simulink model "env_extQ16"  (R2022b)
settings: Solver=VariableStepAuto  StartTime=0.0  StopTime=30  RelTol=1e-3
values from neighbouring files (symbols this model uses):
  B = 8    [variables.m]    (also in variables16.m)
  cordic_delay = 20    [variables.m]    (also in variables16.m)
  e_val = 1/l2    [variables.m]    (also in variables16.m)
  exp_fract_len_homo = 26    [variables.m]    (also in variables16.m = 10)
  exp_word_len_homo = 32    [variables.m]    (also in variables16.m = 16)
  explarge_delay = 3    [variables.m]    (also in variables16.m)
  fft_len_hilb = 2048    [variables.m]    (also in variables16.m)
  fft_length = 4096    [variables.m]    (also in variables16.m)
  frac_bit_l2 = 30    [variables.m]    (also in variables16.m = 14)
  frac_bit_l3 = 29    [variables.m]    (also in variables16.m = 13)
  frac_bit_l4 = 28    [variables.m]    (also in variables16.m = 12)
  grp_delay_hilb = 11    [variables.m]    (also in variables16.m)
  grp_delay_homo = 13    [variables.m]    (also in variables16.m)
  grp_delay_psd = 19    [variables.m]    (also in variables16.m)
  grp_delay_swt = 12    [variables.m]    (also in variables16.m)
  l2 = log(2)    [variables.m]    (also in variables16.m)
  l2e = 1/log2(exp(1))    [variables.m]    (also in variables16.m)
  log2_table = log2((2^(B-1) : 2^(B)) / 2^(B - 1))    [variables.m]    (also in variables16.m)
  log_fract_len_homo = 31    [variables.m]    (also in variables16.m = 15)
  log_latency = 21    [variables.m]    (also in variables16.m)
  log_word_len = 48    [variables.m]    (also in variables16.m = 24)
  log_word_len_homo = 32    [variables.m]    (also in variables16.m = 16)
  NLZLUT = B-ceil(log2((1:2^B)))    [variables.m]    (also in variables16.m)
  scale = 1.0 / (fs * sum(window_val.*window_val))    [variables.m]    (also in variables16.m)
  win_dim = 64    [variables.m]    (also in variables16.m)
  window_dim = 100    [variables.m]    (also in variables16.m)
undefined symbols (not defined in the file or in its folder): C, c, fl_high_index, fl_low_index, HiD, hilbert_fifo_full, LoD, psd_fifo_full, SFVC784, swt_fifo_full, XCK26, xlfda_numerator
libraries: hdlBasic x626, hdlDSPIP x12, hdlUtilities x2, dspsnks4 x1, dspvision x1, vmcUtilities x1
(part 2 of 7)

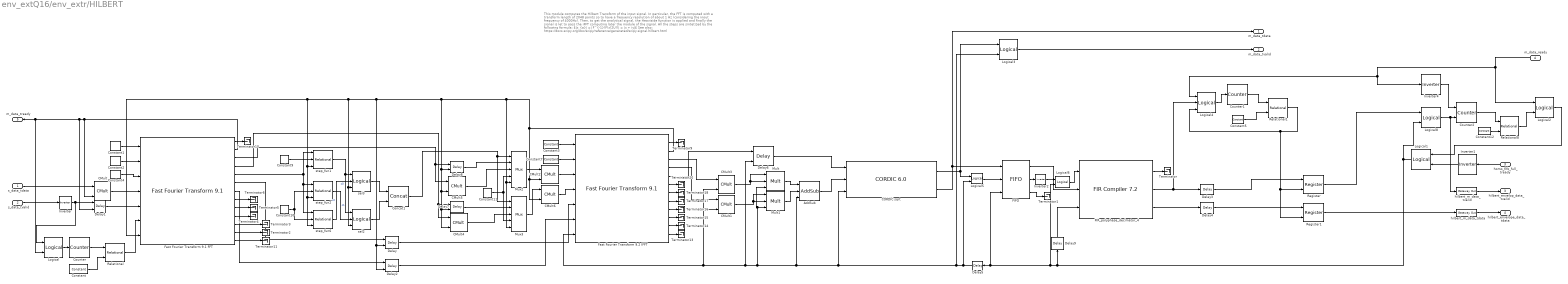
== system env_extQ16/env_extr/HILBERT ==
  note: This module computes the Hilbert Transform of the input signal.
      | In particular, the FFT is computed with a transform length of 2048 points so to have a frequency resolution of about 1 Hz (considering the input frequency of 4000Hz).
      | Then, to get the analytical signal, the Heaviside function is applied and finally the signal is let to pass the iFFT computing later the module of the signal.
      |
      | All the steps are sintetized by the following formula:
      | $|x_{a}| =| F^{-1}(F(x)2U))| = |x + iy|$
      |
      | See also: https://docs.scipy.org/doc/scipy/reference/generated/scipy.signal.hilbert.html
  s_data_tdata : Inport
  s_data_tvalid : Inport  Port=2
  homo_fifo_full_tready : Inport  Port=3
  m_data_ready : Inport  Port=4
  AddSub : hdlBasic/AddSub  mode=Addition  use_carryin=off  use_carryout=off  en=on  latency=1  precision=User Defined  arith_type=Unsigned  n_bits=32  bin_pt=31  quantization="Round  (unbiased: +/- Inf)"  overflow=Wrap  use_behavioral_HDL=off  hw_selection=Fabric  pipelined=off  XmcBlockStatus=1  maskContainerNames=tabcontainer1  block_type=addsub  block_config=sysgen:Addsub_config
  CMult : hdlBasic/CMult  const=1/2  gui_display_data_type=Fixed-point  const_n_bits=32  const_bin_pt=31  float_type=Single  exp_bits=8  fraction_bits=24  en=on  latency=1  precision=User Defined  arith_type="Signed  (2's comp)"  n_bits=34  bin_pt=33  quantization="Round  (unbiased: +/- Inf)"  overflow=Wrap  use_behavioral_HDL=off  mem_type=Distributed RAM  pipeline=off  XmcBlockStatus=1  maskContainerNames=tabcontainer1  block_type=cmult  block_config=sysgen:CMult_config
      settings: infoedit=[]
  CMult1 : hdlBasic/CMult  const=1/fft_len_hilb*128  gui_display_data_type=Fixed-point  const_n_bits=32  const_bin_pt=31  float_type=Single  exp_bits=8  fraction_bits=24  en=on  latency=1  precision=User Defined  arith_type="Signed  (2's comp)"  n_bits=32  bin_pt=30  quantization="Round  (unbiased: +/- Inf)"  overflow=Wrap  use_behavioral_HDL=off  mem_type=Distributed RAM  pipeline=off  XmcBlockStatus=1  maskContainerNames=tabcontainer1  block_type=cmult  block_config=sysgen:CMult_config
      settings: infoedit=[]
  CMult2 : hdlBasic/CMult  const=1/64  gui_display_data_type=Fixed-point  const_n_bits=32  const_bin_pt=31  float_type=Single  exp_bits=8  fraction_bits=24  en=on  latency=1  precision=User Defined  arith_type="Signed  (2's comp)"  n_bits=34  bin_pt=33  quantization="Round  (unbiased: +/- Inf)"  overflow=Wrap  use_behavioral_HDL=off  mem_type=Distributed RAM  pipeline=off  XmcBlockStatus=1  maskContainerNames=tabcontainer1  block_type=cmult  block_config=sysgen:CMult_config
      settings: infoedit=[]
  CMult3 : hdlBasic/CMult  const=1/fft_len_hilb*128  gui_display_data_type=Fixed-point  const_n_bits=32  const_bin_pt=31  float_type=Single  exp_bits=8  fraction_bits=24  en=on  latency=1  precision=User Defined  arith_type="Signed  (2's comp)"  n_bits=32  bin_pt=30  quantization="Round  (unbiased: +/- Inf)"  overflow=Wrap  use_behavioral_HDL=off  mem_type=Distributed RAM  pipeline=off  XmcBlockStatus=1  maskContainerNames=tabcontainer1  block_type=cmult  block_config=sysgen:CMult_config
      settings: infoedit=[]
  CMult4 : hdlBasic/CMult  const=2  gui_display_data_type=Fixed-point  const_n_bits=32  const_bin_pt=30  float_type=Single  exp_bits=8  fraction_bits=24  en=on  latency=2  precision=Full  arith_type="Signed  (2's comp)"  n_bits=16  bin_pt=14  quantization=Truncate  overflow=Wrap  use_behavioral_HDL=off  mem_type=Distributed RAM  pipeline=off  XmcBlockStatus=1  maskContainerNames=tabcontainer1  block_type=cmult  block_config=sysgen:CMult_config
      settings: infoedit=[]
  CMult5 : hdlBasic/CMult  const=2  gui_display_data_type=Fixed-point  const_n_bits=32  const_bin_pt=30  float_type=Single  exp_bits=8  fraction_bits=24  en=on  latency=2  precision=Full  arith_type="Signed  (2's comp)"  n_bits=16  bin_pt=14  quantization=Truncate  overflow=Wrap  use_behavioral_HDL=off  mem_type=Distributed RAM  pipeline=off  XmcBlockStatus=1  maskContainerNames=tabcontainer1  block_type=cmult  block_config=sysgen:CMult_config
      settings: infoedit=[]
  CMult6 : hdlBasic/CMult  const=1/64  gui_display_data_type=Fixed-point  const_n_bits=32  const_bin_pt=31  float_type=Single  exp_bits=8  fraction_bits=24  en=on  latency=1  precision=User Defined  arith_type="Signed  (2's comp)"  n_bits=34  bin_pt=33  quantization="Round  (unbiased: +/- Inf)"  overflow=Wrap  use_behavioral_HDL=off  mem_type=Distributed RAM  pipeline=off  XmcBlockStatus=1  maskContainerNames=tabcontainer1  block_type=cmult  block_config=sysgen:CMult_config
      settings: infoedit=[]
  CORDIC sqrt : hdlDSPIP/CORDIC 6.0   functional_selection=Square_Root  architectural_configuration=Parallel  pipelining_mode=Maximum  data_format=UnsignedFraction  phase_format=Radians  input_width=32  output_width=32  round_mode=Nearest_Even  iterations=0  precision=0  compensation_scaling=No_Scale_Compensation  coarse_rotation=off  aclken=on  aresetn=off  out_tready=off  cartesian_has_tuser=off  cartesian_has_tlast=off  cartesian_tuser_width=1  phase_has_tuser=off  phase_has_tlast=off  phase_tuser_width=1  out_tlast_behv=Null  flow_control=NonBlocking  optimize_goal=Resources  trim_axipin_name=off  simulation_type=hybrid_sim  simulation_model=sysgen:cordic_v6_0  data_path_portlist={'s_axis_cartesian_tdata_imag', 's_axis_cartesian_tdata_real', 's_axis_phase_tdata_phase', 'm_axis_dout_tdata_imag', 'm_axis_dout_tdata_real', 'm_axis_dout_tdata_phase','m_axis_dout_tdata'}  ip_name=CORDIC  ip_version=6.0  dsptool_ready=true  ipcore_usecache=true  ipcore_useipmodelcache=true  wrapper_available=true  port_translation_map={ 'aclken' => 'en', 'aresetn' => 'rst' }  XmcBlockStatus=1  maskContainerNames=group15  block_type=cordic_v6_0  block_config=sysgen:rodinimport_config  block_width=800
  Concat1 : hdlBasic/Concat  num_inputs=2  XmcBlockStatus=1  maskContainerNames=group1  block_type=concat  block_config=sysgen:Concat_config
  Constant : hdlBasic/Constant  const=fft_len_hilb-1  gui_display_data_type=Fixed-point  arith_type=Signed (2's comp)  n_bits=log2(fft_len_hilb)+1  bin_pt=0  preci_type=Single  exp_width=8  frac_width=24  explicit_period=off  period=1  XmcBlockStatus=1  maskContainerNames=tabcontainer1  block_type=constant  block_config=sysgen:Constant_config
  Constant1 : hdlBasic/Constant  const=1.0  gui_display_data_type=Fixed-point  arith_type=Unsigned  n_bits=1  bin_pt=0  preci_type=Single  exp_width=8  frac_width=24  explicit_period=off  period=1  XmcBlockStatus=1  maskContainerNames=tabcontainer1  block_type=constant  block_config=sysgen:Constant_config
  Constant10 : hdlBasic/Constant  const=fft_len_hilb/2  gui_display_data_type=Fixed-point  arith_type=Unsigned  n_bits=ceil(log2(fft_len_hilb/2+1))  bin_pt=0  preci_type=Single  exp_width=8  frac_width=24  explicit_period=on  period=sample_period_hilbert  XmcBlockStatus=1  maskContainerNames=tabcontainer1  block_type=constant  block_config=sysgen:Constant_config
  Constant11 : hdlBasic/Constant  const=0  gui_display_data_type=Fixed-point  arith_type=Signed (2's comp)  n_bits=16  bin_pt=14  preci_type=Single  exp_width=8  frac_width=24  explicit_period=off  period=1  XmcBlockStatus=1  maskContainerNames=tabcontainer1  block_type=constant  block_config=sysgen:Constant_config
  Constant12 : hdlBasic/Constant  const=win_dim  gui_display_data_type=Fixed-point  arith_type=Unsigned  n_bits=win_bit  bin_pt=0  preci_type=Single  exp_width=8  frac_width=24  explicit_period=off  period=1  XmcBlockStatus=1  maskContainerNames=tabcontainer1  block_type=constant  block_config=sysgen:Constant_config
  Constant2 : hdlBasic/Constant  const=1.0  gui_display_data_type=Boolean  arith_type=Boolean  n_bits=1  bin_pt=0  preci_type=Single  exp_width=8  frac_width=24  explicit_period=off  period=1  XmcBlockStatus=1  maskContainerNames=tabcontainer1  block_type=constant  block_config=sysgen:Constant_config
  Constant3 : hdlBasic/Constant  const=0  gui_display_data_type=Fixed-point  arith_type=Unsigned  n_bits=1  bin_pt=0  preci_type=Single  exp_width=8  frac_width=24  explicit_period=off  period=1  XmcBlockStatus=1  maskContainerNames=tabcontainer1  block_type=constant  block_config=sysgen:Constant_config
  Constant4 : hdlBasic/Constant  const=0  gui_display_data_type=Fixed-point  arith_type=Signed (2's comp)  n_bits=34  bin_pt=33  preci_type=Single  exp_width=8  frac_width=24  explicit_period=on  period=sample_period_hilbert  XmcBlockStatus=1  maskContainerNames=tabcontainer1  block_type=constant  block_config=sysgen:Constant_config
  Constant5 : hdlBasic/Constant  const=grp_delay_hilb  gui_display_data_type=Fixed-point  arith_type=Unsigned  n_bits=ceil(log2(grp_delay_hilb))  bin_pt=0  preci_type=Single  exp_width=8  frac_width=24  explicit_period=off  period=1  XmcBlockStatus=1  maskContainerNames=tabcontainer1  block_type=constant  block_config=sysgen:Constant_config
  Constant7 : hdlBasic/Constant  const=1.0  gui_display_data_type=Boolean  arith_type=Boolean  n_bits=1  bin_pt=0  preci_type=Single  exp_width=8  frac_width=24  explicit_period=off  period=1  XmcBlockStatus=1  maskContainerNames=tabcontainer1  block_type=constant  block_config=sysgen:Constant_config
  Constant9 : hdlBasic/Constant  const=0  gui_display_data_type=Fixed-point  arith_type=Unsigned  n_bits=1  bin_pt=0  preci_type=Single  exp_width=8  frac_width=24  explicit_period=on  period=sample_period_hilbert  XmcBlockStatus=1  maskContainerNames=tabcontainer1  block_type=constant  block_config=sysgen:Constant_config
  Counter : hdlBasic/Counter  cnt_type=Free running  cnt_to=Inf  operation=Up  start_count=0  cnt_by_val=1  arith_type=Unsigned  n_bits=11  bin_pt=0  load_pin=off  rst=off  en=on  explicit_period=Explicit  period=sample_period_hilbert  use_behavioral_HDL=off  implementation=Fabric  XmcBlockStatus=1  maskContainerNames=group1  block_type=counter  block_config=sysgen:Counter_config  block_width=531  block_height=1023
  Counter1 : hdlBasic/Counter  cnt_type=Free running  cnt_to=Inf  operation=Up  start_count=0  cnt_by_val=1  arith_type=Unsigned  n_bits=ceil(log2(grp_delay_hilb))  bin_pt=0  load_pin=off  rst=off  en=on  explicit_period=Explicit  period=sample_period_hilbert  use_behavioral_HDL=off  implementation=Fabric  XmcBlockStatus=1  maskContainerNames=group1  block_type=counter  block_config=sysgen:Counter_config  block_width=531  block_height=1023
  Counter2 : hdlBasic/Counter  cnt_type=Free running  cnt_to=Inf  operation=Up  start_count=0  cnt_by_val=1  arith_type=Unsigned  n_bits=win_bit  bin_pt=0  load_pin=off  rst=on  en=on  explicit_period=Explicit  period=sample_period_psd  use_behavioral_HDL=off  implementation=Fabric  XmcBlockStatus=1  maskContainerNames=group1  block_type=counter  block_config=sysgen:Counter_config  block_width=531  block_height=1023
  Delay : hdlBasic/Delay  rst=off  en=on  latency=4  reg_retiming=off  XmcBlockStatus=1  maskContainerNames=group1  block_type=delay  block_config=sysgen:Delay_config
  Delay1 : hdlBasic/Delay  rst=off  en=on  latency=1  reg_retiming=off  XmcBlockStatus=1  maskContainerNames=group1  block_type=delay  block_config=sysgen:Delay_config
  Delay2 : hdlBasic/Delay  rst=off  en=on  latency=4  reg_retiming=off  XmcBlockStatus=1  maskContainerNames=group1  block_type=delay  block_config=sysgen:Delay_config
  Delay3 : hdlBasic/Delay  rst=off  en=off  latency=1  reg_retiming=off  XmcBlockStatus=1  maskContainerNames=group1  block_type=delay  block_config=sysgen:Delay_config
  Delay4 : hdlBasic/Delay  rst=off  en=off  latency=1  reg_retiming=off  XmcBlockStatus=1  maskContainerNames=group1  block_type=delay  block_config=sysgen:Delay_config
  Delay5 : hdlBasic/Delay  rst=off  en=off  latency=64*(grp_delay_homo-grp_delay_hilb)  reg_retiming=off  XmcBlockStatus=1  maskContainerNames=group1  block_type=delay  block_config=sysgen:Delay_config
  Delay6 : hdlBasic/Delay  rst=off  en=on  latency=5  reg_retiming=off  XmcBlockStatus=1  maskContainerNames=group1  block_type=delay  block_config=sysgen:Delay_config
  Delay7 : hdlBasic/Delay  rst=off  en=on  latency=2  reg_retiming=off  XmcBlockStatus=1  maskContainerNames=group1  block_type=delay  block_config=sysgen:Delay_config
  Delay8 : hdlBasic/Delay  rst=off  en=on  latency=2  reg_retiming=off  XmcBlockStatus=1  maskContainerNames=group1  block_type=delay  block_config=sysgen:Delay_config
  Delay9 : hdlBasic/Delay  rst=off  en=off  latency=1  reg_retiming=off  XmcBlockStatus=1  maskContainerNames=group1  block_type=delay  block_config=sysgen:Delay_config
  FIFO : hdlBasic/FIFO  mem_type=Block RAM  performance_options=Standard_FIFO  embedded_registers=off  depth=256  use_asym_data_widths=off  asym_read_width=32  percent_nbits=1  rst=off  rst_latency=2  en=off  use_dcount=off  use_percent_full_port=off  use_almost_empty=off  almost_empty_thresh=2  use_almost_full=off  use_rd_rst_busy=off  use_wr_rst_busy=off  almost_full_thresh=14  almost_empty_offset=[]  almost_full_offset=[]  explicit_period=off  period=[]  store_only_valid=[]  init_zero=[]  simulation_type=fast_sim  XmcBlockStatus=1  maskContainerNames=tabcontainer1  block_type=fifo  block_config=sysgen:FIFO_config  block_width=538  block_height=997
      settings: infoedit=[]
  FIR_polyphase_decimator_4 : hdlDSPIP/FIR Compiler 7.2   coefficientvector=firdecim.Numerator  coefficient_sets=1  coefficient_reload=off  filter_type=Decimation  rate_change_type=Integer  interpolation_rate=1  decimation_rate=80  zero_pack_factor=1  channel_sequence=Basic  number_channels=1  pattern_list='P4-0,P4-1,P4-2,P4-3,P4-4'  number_paths=1  ratespecification=Input_Sample_Period  sampleperiod=1.00000000  hardwareoversamplingrate=1  coefficient_sign=Signed  quantization=Quantize_Only  coefficient_width=coeff_width  bestprecision=on  coefficient_fractional_bits=37  coefficient_structure=Non_Symmetric  output_rounding_mode=Convergent_Rounding_to_Even  output_width=32  filter_architecture=Systolic_Multiply_Accumulate  optimization_goal=Area  optimization_list='None'  data_buffer_type=Automatic  coefficient_buffer_type=Automatic  input_buffer_type=Automatic  output_buffer_type=Automatic  preference_for_other_storage=Automatic  multi_column_support=Automatic  columnconfig='24'  inter_column_pipe_length=4  data_has_tlast=Not_Required  m_data_has_tready=off  s_data_has_fifo=off  s_data_has_tuser=Not_Required  m_data_has_tuser=Not_Required  s_config_sync_mode=On_Vector  s_config_method=Single  num_reload_slots=1  has_aclken=on  has_aresetn=off  reset_data_vector=on  trim_axipin_name=off  simulation_type=hybrid_sim  simulation_model=sysgen:xfirv7_2_cmodel  data_path_portlist={ 's_axis_data_tdata', 'm_axis_data_tdata' }  passband_min=0.0  passband_max=0.5  stopband_min=0.5  stopband_max=1.0  filter_selection=1  gui_behaviour='Sysgen_GUI'  data_sign=Signed  data_width=16  data_fractional_bits=0  data_tuser_width=1  wrapper_available=true  ip_wrap_arbitrary_binary_point=true  ip_name=FIR Compiler  ip_version=7.2  dsptool_ready=true  ipcore_usecache=true  ipcore_useipmodelcache=true  port_translation_map={ 'aclken' => 'en', 'aresetn' => 'rst' }  run_core_at_system_period=true  ipcore_xco_need_fpga_part=true  ipcore_fpga_part=[]  XmcBlockStatus=1  maskContainerNames=tabcontainer1  block_type=fir_compiler_v7_2  block_config=sysgen:rodinimport_config  block_width=820  block_height=600
  Fast Fourier Transform 9.1 FFT : hdlDSPIP/Fast Fourier Transform 9.1   transform_length=2048  target_clock_frequency=fft_freq  target_data_throughput=50  implementation_options=radix_2_burst_io  run_time_configurable_transform_length=off  phase_factor_width=33  scaling_options=unscaled  rounding_modes=convergent_rounding  aclken=off  aresetn=off  output_ordering=natural_order  cyclic_prefix_insertion=off  throttle_scheme=nonrealtime  xk_index=on  ovflo=off  trim_axipin_name=off  memory_options_data=block_ram  memory_options_phase_factors=block_ram  number_of_stages_using_block_ram_for_data_and_phase_factors=6  memory_options_reorder=block_ram  memory_options_hybrid=off  complex_mult_type=use_mults_resources  butterfly_type=use_luts  simulation_type=hybrid_sim  simulation_model=sysgen:xfftv9_cmodel  data_path_portlist={ 's_axis_data_tdata', 'm_axis_data_tdata', 'm_axis_status_tdata', 'event_fft_overflow' }  channels=1  input_ordering=natural_order  input_width=16  ip_name=Fast Fourier Transform  ip_version=9.1  dsptool_ready=true  ipcore_usecache=true  ipcore_useipmodelcache=true  wrapper_available=true  port_translation_map={ 'aclken' => 'en', 'aresetn' => 'rst'}  data_format=fixed_point  XmcBlockStatus=1  maskContainerNames=tabcontainer1  block_type=xfft_v9_1  block_config=sysgen:rodinimport_config
  Fast Fourier Transform 9.2 IFFT : hdlDSPIP/Fast Fourier Transform 9.1   transform_length=2048  target_clock_frequency=fft_freq  target_data_throughput=50  implementation_options=radix_2_burst_io  run_time_configurable_transform_length=off  phase_factor_width=33  scaling_options=unscaled  rounding_modes=convergent_rounding  aclken=off  aresetn=off  output_ordering=natural_order  cyclic_prefix_insertion=off  throttle_scheme=nonrealtime  xk_index=off  ovflo=off  trim_axipin_name=off  memory_options_data=block_ram  memory_options_phase_factors=block_ram  number_of_stages_using_block_ram_for_data_and_phase_factors=6  memory_options_reorder=block_ram  memory_options_hybrid=off  complex_mult_type=use_mults_resources  butterfly_type=use_luts  simulation_type=hybrid_sim  simulation_model=sysgen:xfftv9_cmodel  data_path_portlist={ 's_axis_data_tdata', 'm_axis_data_tdata', 'm_axis_status_tdata', 'event_fft_overflow' }  channels=1  input_ordering=natural_order  input_width=16  ip_name=Fast Fourier Transform  ip_version=9.1  dsptool_ready=true  ipcore_usecache=true  ipcore_useipmodelcache=true  wrapper_available=true  port_translation_map={ 'aclken' => 'en', 'aresetn' => 'rst'}  data_format=fixed_point  XmcBlockStatus=1  maskContainerNames=tabcontainer1  block_type=xfft_v9_1  block_config=sysgen:rodinimport_config
  Inverter{,1..2,4} (4 alike) : hdlBasic/Inverter  en=off  latency=0  XmcBlockStatus=1  maskContainerNames=group2  block_type=inv  block_config=sysgen:Inverter_config
  Logical{,1..3,5..6,8} (7 alike) : hdlBasic/Logical  logical_function=AND  inputs=2  en=off  latency=0  precision=Full  arith_type=Unsigned  n_bits=16  bin_pt=0  align_bp=on  overflow=[]  quantization=[]  XmcBlockStatus=1  maskContainerNames=tabcontainer1  block_type=logical  block_config=sysgen:Logical_config
  Logical4 : hdlBasic/Logical  logical_function=AND  inputs=3  en=off  latency=0  precision=Full  arith_type=Unsigned  n_bits=16  bin_pt=0  align_bp=on  overflow=[]  quantization=[]  XmcBlockStatus=1  maskContainerNames=tabcontainer1  block_type=logical  block_config=sysgen:Logical_config
  Mult : hdlBasic/Mult  precision=User Defined  arith_type="Signed  (2's comp)"  n_bits=32  bin_pt=31  quantization="Round  (unbiased: +/- Inf)"  overflow=Wrap  en=on  latency=3  use_behavioral_HDL=off  opt=Speed  use_embedded=on  optimum_pipeline=off  pipeline=on  use_rpm=on  placement_style=Triangular  XmcBlockStatus=1  maskContainerNames=group1  block_type=mult  block_config=sysgen:Mult_config  block_width=598  block_height=876
  Mult1 : hdlBasic/Mult  precision=User Defined  arith_type="Signed  (2's comp)"  n_bits=32  bin_pt=31  quantization="Round  (unbiased: +/- Inf)"  overflow=Wrap  en=on  latency=3  use_behavioral_HDL=off  opt=Speed  use_embedded=on  optimum_pipeline=off  pipeline=on  use_rpm=on  placement_style=Triangular  XmcBlockStatus=1  maskContainerNames=group1  block_type=mult  block_config=sysgen:Mult_config  block_width=598  block_height=876
  Mux2 : hdlBasic/Mux  inputs=3  en=on  latency=1  precision=Full  arith_type="Signed  (2's comp)"  n_bits=34  bin_pt=26  quantization="Round  (unbiased: +/- Inf)"  overflow=Wrap  XmcBlockStatus=1  maskContainerNames=tabcontainer1  block_type=mux  block_config=sysgen:Mux_config
  Mux3 : hdlBasic/Mux  inputs=3  en=on  latency=1  precision=Full  arith_type="Signed  (2's comp)"  n_bits=34  bin_pt=26  quantization="Round  (unbiased: +/- Inf)"  overflow=Wrap  XmcBlockStatus=1  maskContainerNames=tabcontainer1  block_type=mux  block_config=sysgen:Mux_config
  Register : hdlBasic/Register  init=0  rst=on  en=off  XmcBlockStatus=1  maskContainerNames=tabcontainer1  block_type=register  block_config=sysgen:Register_config
  Register1 : hdlBasic/Register  init=0  rst=on  en=off  XmcBlockStatus=1  maskContainerNames=tabcontainer1  block_type=register  block_config=sysgen:Register_config
  Relational : hdlBasic/Relational  mode=a=b  op_type=Bool  en=off  latency=1  XmcBlockStatus=1  maskContainerNames=tabcontainer1  block_type=relational  block_config=sysgen:Relational_config
  Relational1 : hdlBasic/Relational  mode=a<b  op_type=Bool  en=off  latency=0  XmcBlockStatus=1  maskContainerNames=tabcontainer1  block_type=relational  block_config=sysgen:Relational_config
  Relational8 : hdlBasic/Relational  mode=a<b  op_type=Bool  en=off  latency=0  XmcBlockStatus=1  maskContainerNames=tabcontainer1  block_type=relational  block_config=sysgen:Relational_config
  Terminator{,1..6,9..11,13..18,20} (17 alike) : Terminator
  hilbert_m_data_tdata : hdlBasic/Gateway Out  inherit_from_input=off  hdl_port=on  rows=1  columns=1  UseAsDAC=off  DACChannel='1'  interface=None  automatic_assignment=on  address_offset=hex2dec('00')  intf_name=''  intf_description=''  timing_constraint=None  locs_specified=off  LOCs={}  io_standard={}  XmcBlockStatus=1  maskContainerNames=group4  block_type=gatewayout  block_config=sysgen:gateway_out_config  block_width_w=590  block_height_w=620  block_width=620  block_height=750
  hilbert_m_data_tvalid : hdlBasic/Gateway Out  inherit_from_input=off  hdl_port=on  rows=1  columns=1  UseAsDAC=off  DACChannel='1'  interface=None  automatic_assignment=on  address_offset=hex2dec('00')  intf_name=''  intf_description=''  timing_constraint=None  locs_specified=off  LOCs={}  io_standard={}  XmcBlockStatus=1  maskContainerNames=group4  block_type=gatewayout  block_config=sysgen:gateway_out_config  block_width_w=590  block_height_w=620  block_width=620  block_height=750
  sel2 : hdlBasic/Logical  logical_function=AND  inputs=2  en=on  latency=1  precision=Full  arith_type=Unsigned  n_bits=16  bin_pt=0  align_bp=on  overflow=[]  quantization=[]  XmcBlockStatus=1  maskContainerNames=tabcontainer1  block_type=logical  block_config=sysgen:Logical_config
  sel3 : hdlBasic/Logical  logical_function=AND  inputs=2  en=on  latency=1  precision=Full  arith_type=Unsigned  n_bits=16  bin_pt=0  align_bp=on  overflow=[]  quantization=[]  XmcBlockStatus=1  maskContainerNames=tabcontainer1  block_type=logical  block_config=sysgen:Logical_config
  step_fun1 : hdlBasic/Relational  mode=a!=b  op_type=Bool  en=on  latency=1  XmcBlockStatus=1  maskContainerNames=tabcontainer1  block_type=relational  block_config=sysgen:Relational_config
  step_fun2 : hdlBasic/Relational  mode=a<b  op_type=Bool  en=on  latency=1  XmcBlockStatus=1  maskContainerNames=tabcontainer1  block_type=relational  block_config=sysgen:Relational_config
  step_fun6 : hdlBasic/Relational  mode=a>b  op_type=Bool  en=on  latency=1  XmcBlockStatus=1  maskContainerNames=tabcontainer1  block_type=relational  block_config=sysgen:Relational_config
  m_data_tdata : Outport
  m_data_tvalid : Outport  Port=2
  hilbert_envelop_data_tvalid : Outport  Port=3
  hilbert_envelope_data_tdata : Outport  Port=4
  m_data_tready : Outport  Port=5
  wires:
  Constant4/1 -> Fast Fourier Transform 9.1 FFT/3
  Constant1/1 -> Fast Fourier Transform 9.1 FFT/1
  Fast Fourier Transform 9.1 FFT/9 -> Terminator5/1
  Fast Fourier Transform 9.1 FFT/8 -> Terminator6/1
  Fast Fourier Transform 9.1 FFT/10 -> Terminator4/1
  Fast Fourier Transform 9.1 FFT/12 -> Terminator2/1
  Fast Fourier Transform 9.1 FFT/1 -> Terminator10/1
  Fast Fourier Transform 9.1 FFT/13 -> Terminator11/1
  Relational/1 -> Fast Fourier Transform 9.1 FFT/6
  Fast Fourier Transform 9.2 IFFT/10 -> Terminator15/1
  Fast Fourier Transform 9.2 IFFT/11 -> Terminator14/1
  Fast Fourier Transform 9.2 IFFT/12 -> Terminator13/1
  Constant7/1 -> Fast Fourier Transform 9.2 IFFT/2
  Fast Fourier Transform 9.2 IFFT/1 -> Terminator9/1
  Fast Fourier Transform 9.2 IFFT/7 -> Terminator18/1
  Delay/1 -> Fast Fourier Transform 9.2 IFFT/5
  Fast Fourier Transform 9.2 IFFT/5 -> Delay6/1
  Fast Fourier Transform 9.2 IFFT/6 -> Terminator20/1
  Fast Fourier Transform 9.2 IFFT/4 -> CMult1/1
  CMult3/1 -> Mult/2, Mult/1
  Fast Fourier Transform 9.2 IFFT/3 -> CMult3/1
  Constant11/1 -> Mux2/4, Mux3/4
  Delay7/1 -> Mux3/2
  CMult5/1 -> Mux2/3
  Delay8/1 -> Mux2/2
  CMult4/1 -> Mux3/3
  Mux3/1 -> CMult6/1
  Mux2/1 -> CMult2/1
  sel2/1 -> Concat1/2
  step_fun1/1 -> sel2/1, sel3/1  "c0"
  Constant10/1 -> step_fun2/2, step_fun6/2
  step_fun6/1 -> sel3/2  "c2"
  sel3/1 -> Concat1/1
  Constant9/1 -> step_fun1/2
  Fast Fourier Transform 9.1 FFT/5 -> step_fun6/1, step_fun2/1, step_fun1/1
  step_fun2/1 -> sel2/2  "c1"
  Concat1/1 -> Mux2/1, Mux3/1
  hilbert_m_data_tdata/1 -> hilbert_envelope_data_tdata/1
  Constant2/1 -> Fast Fourier Transform 9.1 FFT/2
  s_data_tdata/1 -> CMult/1
  Constant3/1 -> Fast Fourier Transform 9.2 IFFT/1
  s_data_tvalid/1 -> Inverter/1
  CMult6/1 -> Fast Fourier Transform 9.2 IFFT/4
  CMult2/1 -> Fast Fourier Transform 9.2 IFFT/3
  FIR_polyphase_decimator_4/2 -> Logical4/2, Delay3/1
  FIR_polyphase_decimator_4/3 -> Delay4/1
  Delay2/1 -> Fast Fourier Transform 9.2 IFFT/6
  Fast Fourier Transform 9.1 FFT/7 -> Delay2/1
  Counter/1 -> Relational/1
  Constant/1 -> Relational/2
  Logical/1 -> Counter/1
  Fast Fourier Transform 9.2 IFFT/8 -> Terminator17/1
  Fast Fourier Transform 9.2 IFFT/9 -> Terminator16/1
  CMult1/1 -> Mult1/1, Mult1/2
  Mult/1 -> AddSub/1
  Mult1/1 -> AddSub/2
  homo_fifo_full_tready/1 -> Inverter1/1
  AddSub/1 -> CORDIC sqrt/2
  Delay6/1 -> CORDIC sqrt/1
  CMult/1 -> Fast Fourier Transform 9.1 FFT/4
  Delay1/1 -> Fast Fourier Transform 9.1 FFT/5
  Inverter/1 -> Logical/1, Delay1/1
  Counter2/1 -> Relational8/1
  Inverter4/1 -> Counter2/1
  Constant12/1 -> Relational8/2
  hilbert_m_data_tvalid/1 -> hilbert_envelop_data_tvalid/1
  Logical8/1 -> hilbert_m_data_tvalid/1, Counter2/2
  CORDIC sqrt/1 -> Logical3/1, Logical5/1
  m_data_ready/1 -> Logical4/1, Inverter4/1, Logical2/1
  Fast Fourier Transform 9.2 IFFT/2 -> CMult6/2, CMult2/2, Mux3/5, Mux2/5, CMult4/2, Delay7/2, CMult5/2, Delay8/2, Delay2/2, Delay/2, sel2/3, sel3/3, step_fun2/3, step_fun6/3, step_fun1/3, Fast Fourier Transform 9.1 FFT/7
  Logical1/1 -> Logical8/2, Delay5/1, FIFO/3, Logical6/2, Delay9/1
  Fast Fourier Transform 9.1 FFT/2 -> m_data_tready/1, Logical/2, Delay1/2, CMult/2
  Fast Fourier Transform 9.1 FFT/6 -> Delay/1
  Fast Fourier Transform 9.1 FFT/4 -> CMult4/1, Delay7/1
  Fast Fourier Transform 9.1 FFT/3 -> CMult5/1, Delay8/1
  Fast Fourier Transform 9.1 FFT/11 -> Terminator3/1
  Inverter1/1 -> Logical1/2
  Logical3/1 -> m_data_tvalid/1
  CORDIC sqrt/2 -> m_data_tdata/1, FIFO/1
  Relational8/1 -> Logical2/2
  Logical2/1 -> Logical1/1
  FIR_polyphase_decimator_4/1 -> Terminator/1
  Counter1/1 -> Relational1/1
  Logical4/1 -> Counter1/1
  Relational1/1 -> Register/2, Register1/2, Logical4/3
  Constant5/1 -> Relational1/2
  Delay3/1 -> Register/1
  Delay4/1 -> Register1/1
  Register/1 -> Logical8/1
  Register1/1 -> hilbert_m_data_tdata/1
  FIFO/2 -> Inverter2/1
  FIFO/3 -> Terminator1/1
  Delay5/1 -> Logical5/2, Logical3/2, CORDIC sqrt/3, AddSub/3, Mult/3, Mult1/3, Delay6/2, Fast Fourier Transform 9.2 IFFT/7, CMult1/2, CMult3/2
  Delay9/1 -> FIR_polyphase_decimator_4/3
  Logical5/1 -> FIFO/2
  FIFO/1 -> FIR_polyphase_decimator_4/2
  Inverter2/1 -> Logical6/1
  Logical6/1 -> FIR_polyphase_decimator_4/1

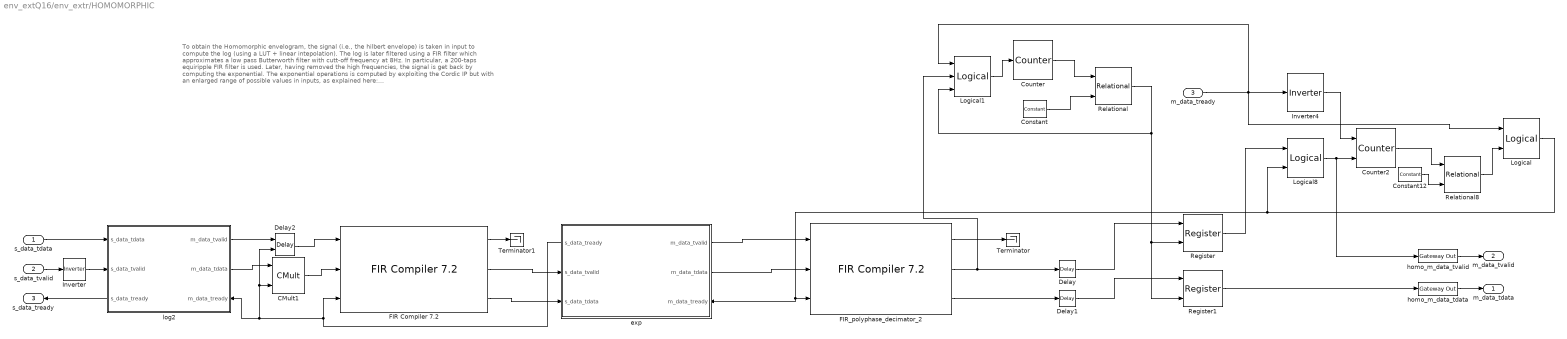
== system env_extQ16/env_extr/HOMOMORPHIC ==
  note: To obtain the Homomorphic envelogram, the signal (i.e., the hilbert envelope) is taken in input to compute the log (using a LUT + linear intepolation).
      |
      | The log is later filtered using a FIR filter which approximates a low pass Butterworth filter with cutt-off frequency at 8Hz. In particular, a 200-taps equiripple FIR filter is used.
      |
      | Later, having removed the high frequencies, the signal is get back by computing the exponential. The exponential operations is computed by exploiting the Cordic IP but with an enlarged range of possible values in inputs, as explained here: https://ieeexplore.ieee.org/document/9012611 .
  s_data_tdata : Inport
  s_data_tvalid : Inport  Port=2
  m_data_tready : Inport  Port=3
  CMult1 : hdlBasic/CMult  const=l2e  gui_display_data_type=Fixed-point  const_n_bits=32  const_bin_pt=31  float_type=Single  exp_bits=8  fraction_bits=24  en=on  latency=1  precision=User Defined  arith_type="Signed  (2's comp)"  n_bits=32  bin_pt=26  quantization="Round  (unbiased: +/- Inf)"  overflow=Saturate  use_behavioral_HDL=off  mem_type=Distributed RAM  pipeline=off  XmcBlockStatus=1  maskContainerNames=tabcontainer1  block_type=cmult  block_config=sysgen:CMult_config
      settings: infoedit=[]
  Constant : hdlBasic/Constant  const=grp_delay_homo  gui_display_data_type=Fixed-point  arith_type=Unsigned  n_bits=ceil(log2(grp_delay_homo))  bin_pt=0  preci_type=Single  exp_width=8  frac_width=24  explicit_period=off  period=1  XmcBlockStatus=1  maskContainerNames=tabcontainer1  block_type=constant  block_config=sysgen:Constant_config
  Constant12 : hdlBasic/Constant  const=win_dim  gui_display_data_type=Fixed-point  arith_type=Unsigned  n_bits=win_bit  bin_pt=0  preci_type=Single  exp_width=8  frac_width=24  explicit_period=off  period=1  XmcBlockStatus=1  maskContainerNames=tabcontainer1  block_type=constant  block_config=sysgen:Constant_config
  Counter : hdlBasic/Counter  cnt_type=Free running  cnt_to=Inf  operation=Up  start_count=0  cnt_by_val=1  arith_type=Unsigned  n_bits=ceil(log2(grp_delay_homo))  bin_pt=0  load_pin=off  rst=off  en=on  explicit_period=Explicit  period=sample_period_homo  use_behavioral_HDL=off  implementation=Fabric  XmcBlockStatus=1  maskContainerNames=group1  block_type=counter  block_config=sysgen:Counter_config  block_width=531  block_height=1023
  Counter2 : hdlBasic/Counter  cnt_type=Free running  cnt_to=Inf  operation=Up  start_count=0  cnt_by_val=1  arith_type=Unsigned  n_bits=win_bit  bin_pt=0  load_pin=off  rst=on  en=on  explicit_period=Explicit  period=sample_period_psd  use_behavioral_HDL=off  implementation=Fabric  XmcBlockStatus=1  maskContainerNames=group1  block_type=counter  block_config=sysgen:Counter_config  block_width=531  block_height=1023
  Delay : hdlBasic/Delay  rst=off  en=off  latency=1  reg_retiming=off  XmcBlockStatus=1  maskContainerNames=group1  block_type=delay  block_config=sysgen:Delay_config
  Delay1 : hdlBasic/Delay  rst=off  en=off  latency=1  reg_retiming=off  XmcBlockStatus=1  maskContainerNames=group1  block_type=delay  block_config=sysgen:Delay_config
  Delay2 : hdlBasic/Delay  rst=off  en=on  latency=1  reg_retiming=off  XmcBlockStatus=1  maskContainerNames=group1  block_type=delay  block_config=sysgen:Delay_config
  FIR Compiler 7.2 : hdlDSPIP/FIR Compiler 7.2   coefficientvector=NUM  coefficient_sets=1  coefficient_reload=off  filter_type=Single_Rate  rate_change_type=Integer  interpolation_rate=1  decimation_rate=1  zero_pack_factor=1  channel_sequence=Basic  number_channels=1  pattern_list='P4-0,P4-1,P4-2,P4-3,P4-4'  number_paths=1  ratespecification=Input_Sample_Period  sampleperiod=1  hardwareoversamplingrate=1  coefficient_sign=Signed  quantization=Quantize_Only  coefficient_width=coeff_width  bestprecision=on  coefficient_fractional_bits=36  coefficient_structure=Symmetric  output_rounding_mode=Convergent_Rounding_to_Even  output_width=output_width  filter_architecture=Systolic_Multiply_Accumulate  optimization_goal=Area  optimization_list='None'  data_buffer_type=Automatic  coefficient_buffer_type=Automatic  input_buffer_type=Automatic  output_buffer_type=Automatic  preference_for_other_storage=Automatic  multi_column_support=Automatic  columnconfig='91'  inter_column_pipe_length=4  data_has_tlast=Not_Required  m_data_has_tready=off  s_data_has_fifo=off  s_data_has_tuser=Not_Required  m_data_has_tuser=Not_Required  s_config_sync_mode=On_Vector  s_config_method=Single  num_reload_slots=1  has_aclken=on  has_aresetn=off  reset_data_vector=on  trim_axipin_name=off  simulation_type=hybrid_sim  simulation_model=sysgen:xfirv7_2_cmodel  data_path_portlist={ 's_axis_data_tdata', 'm_axis_data_tdata' }  passband_min=0.0  passband_max=0.5  stopband_min=0.5  stopband_max=1.0  filter_selection=1  gui_behaviour='Sysgen_GUI'  data_sign=Signed  data_width=16  data_fractional_bits=0  data_tuser_width=1  wrapper_available=true  ip_wrap_arbitrary_binary_point=true  ip_name=FIR Compiler  ip_version=7.2  dsptool_ready=true  ipcore_usecache=true  ipcore_useipmodelcache=true  port_translation_map={ 'aclken' => 'en', 'aresetn' => 'rst' }  run_core_at_system_period=true  ipcore_xco_need_fpga_part=true  ipcore_fpga_part=[]  XmcBlockStatus=1  maskContainerNames=tabcontainer1  block_type=fir_compiler_v7_2  block_config=sysgen:rodinimport_config  block_width=820  block_height=600
  FIR_polyphase_decimator_2 : hdlDSPIP/FIR Compiler 7.2   coefficientvector=firdecim.Numerator  coefficient_sets=1  coefficient_reload=off  filter_type=Decimation  rate_change_type=Integer  interpolation_rate=1  decimation_rate=80  zero_pack_factor=1  channel_sequence=Basic  number_channels=1  pattern_list='P4-0,P4-1,P4-2,P4-3,P4-4'  number_paths=1  ratespecification=Input_Sample_Period  sampleperiod=1.00000000  hardwareoversamplingrate=1  coefficient_sign=Signed  quantization=Quantize_Only  coefficient_width=coeff_width  bestprecision=on  coefficient_fractional_bits=37  coefficient_structure=Non_Symmetric  output_rounding_mode=Non_Symmetric_Rounding_Down  output_width=output_width  filter_architecture=Systolic_Multiply_Accumulate  optimization_goal=Area  optimization_list='None'  data_buffer_type=Automatic  coefficient_buffer_type=Automatic  input_buffer_type=Automatic  output_buffer_type=Automatic  preference_for_other_storage=Automatic  multi_column_support=Automatic  columnconfig='24'  inter_column_pipe_length=4  data_has_tlast=Not_Required  m_data_has_tready=off  s_data_has_fifo=off  s_data_has_tuser=Not_Required  m_data_has_tuser=Not_Required  s_config_sync_mode=On_Vector  s_config_method=Single  num_reload_slots=1  has_aclken=on  has_aresetn=off  reset_data_vector=on  trim_axipin_name=off  simulation_type=hybrid_sim  simulation_model=sysgen:xfirv7_2_cmodel  data_path_portlist={ 's_axis_data_tdata', 'm_axis_data_tdata' }  passband_min=0.0  passband_max=0.5  stopband_min=0.5  stopband_max=1.0  filter_selection=1  gui_behaviour='Sysgen_GUI'  data_sign=Signed  data_width=16  data_fractional_bits=0  data_tuser_width=1  wrapper_available=true  ip_wrap_arbitrary_binary_point=true  ip_name=FIR Compiler  ip_version=7.2  dsptool_ready=true  ipcore_usecache=true  ipcore_useipmodelcache=true  port_translation_map={ 'aclken' => 'en', 'aresetn' => 'rst' }  run_core_at_system_period=true  ipcore_xco_need_fpga_part=true  ipcore_fpga_part=[]  XmcBlockStatus=1  maskContainerNames=tabcontainer1  block_type=fir_compiler_v7_2  block_config=sysgen:rodinimport_config  block_width=820  block_height=600
  Inverter : hdlBasic/Inverter  en=off  latency=0  XmcBlockStatus=1  maskContainerNames=group2  block_type=inv  block_config=sysgen:Inverter_config
  Inverter4 : hdlBasic/Inverter  en=off  latency=0  XmcBlockStatus=1  maskContainerNames=group2  block_type=inv  block_config=sysgen:Inverter_config
  Logical : hdlBasic/Logical  logical_function=AND  inputs=2  en=off  latency=0  precision=Full  arith_type=Unsigned  n_bits=16  bin_pt=0  align_bp=on  overflow=[]  quantization=[]  XmcBlockStatus=1  maskContainerNames=tabcontainer1  block_type=logical  block_config=sysgen:Logical_config
  Logical1 : hdlBasic/Logical  logical_function=AND  inputs=3  en=off  latency=0  precision=Full  arith_type=Unsigned  n_bits=16  bin_pt=0  align_bp=on  overflow=[]  quantization=[]  XmcBlockStatus=1  maskContainerNames=tabcontainer1  block_type=logical  block_config=sysgen:Logical_config
  Logical8 : hdlBasic/Logical  logical_function=AND  inputs=2  en=off  latency=0  precision=Full  arith_type=Unsigned  n_bits=16  bin_pt=0  align_bp=on  overflow=[]  quantization=[]  XmcBlockStatus=1  maskContainerNames=tabcontainer1  block_type=logical  block_config=sysgen:Logical_config
  Register : hdlBasic/Register  init=0  rst=on  en=off  XmcBlockStatus=1  maskContainerNames=tabcontainer1  block_type=register  block_config=sysgen:Register_config
  Register1 : hdlBasic/Register  init=0  rst=on  en=off  XmcBlockStatus=1  maskContainerNames=tabcontainer1  block_type=register  block_config=sysgen:Register_config
  Relational : hdlBasic/Relational  mode=a<b  op_type=Bool  en=off  latency=0  XmcBlockStatus=1  maskContainerNames=tabcontainer1  block_type=relational  block_config=sysgen:Relational_config
  Relational8 : hdlBasic/Relational  mode=a<b  op_type=Bool  en=off  latency=0  XmcBlockStatus=1  maskContainerNames=tabcontainer1  block_type=relational  block_config=sysgen:Relational_config
  Terminator : Terminator
  Terminator1 : Terminator
  exp : Subsystem
      settings: PortSchema="{\"entries\":[{\"content\":{\"sides\":[{\"content\":{\"connectorIds\":[\"Out3\",\"In1\",\"In2\"]},\"type\":\"ConnectorPlacement.EquallySpacedRectSide\",\"uuid\":\"9d039a16-3a48-49d5-80b7-ade04a8e7f96\"},{\"content\":{\"connectorIds\":[\"Out1\",\"Out2\",\"In3\"],\"side\":\"RIGHT\"},\"type\":\"ConnectorPlacement.EquallySpacedRectSide\",\"uuid\":\"bb4be220-296c-4d2d-b90e-a958a467eb47\"},{\"content\":{\"connectorIds\":[],\"side\":\"TOP\"},\"type\":\"ConnectorPlacement.EquallySpacedRectSide\",\"uuid\":\"bb4a24ca-25c4-4b34-8f6b-74df8c85655a\"}]},\"type\":\"ConnectorPlacement.EquallySpacedConnector\",\"uuid\":\"a2ca7259-7cd6-4f5b-b082-7ba40fce56a8\"}],\"packageUris\":[\"http://schema.mathworks.com/mf0/Connector/R2020b\"],\"version\":\"1.0\"}"
  homo_m_data_tdata : hdlBasic/Gateway Out  inherit_from_input=off  hdl_port=on  rows=1  columns=1  UseAsDAC=off  DACChannel='1'  interface=None  automatic_assignment=on  address_offset=hex2dec('00')  intf_name=''  intf_description=''  timing_constraint=None  locs_specified=off  LOCs={}  io_standard={}  XmcBlockStatus=1  maskContainerNames=group4  block_type=gatewayout  block_config=sysgen:gateway_out_config  block_width_w=590  block_height_w=620  block_width=620  block_height=750
  homo_m_data_tvalid : hdlBasic/Gateway Out  inherit_from_input=off  hdl_port=on  rows=1  columns=1  UseAsDAC=off  DACChannel='1'  interface=None  automatic_assignment=on  address_offset=hex2dec('00')  intf_name=''  intf_description=''  timing_constraint=None  locs_specified=off  LOCs={}  io_standard={}  XmcBlockStatus=1  maskContainerNames=group4  block_type=gatewayout  block_config=sysgen:gateway_out_config  block_width_w=590  block_height_w=620  block_width=620  block_height=750
  log2 : Subsystem
      settings: PortSchema="{\"entries\":[{\"content\":{\"sides\":[{\"content\":{\"connectorIds\":[\"In1\",\"In2\",\"Out3\"]},\"type\":\"ConnectorPlacement.EquallySpacedRectSide\",\"uuid\":\"9d039a16-3a48-49d5-80b7-ade04a8e7f96\"},{\"content\":{\"connectorIds\":[\"Out1\",\"Out2\",\"In3\"],\"side\":\"RIGHT\"},\"type\":\"ConnectorPlacement.EquallySpacedRectSide\",\"uuid\":\"bb4be220-296c-4d2d-b90e-a958a467eb47\"},{\"content\":{\"connectorIds\":[],\"side\":\"TOP\"},\"type\":\"ConnectorPlacement.EquallySpacedRectSide\",\"uuid\":\"bb4a24ca-25c4-4b34-8f6b-74df8c85655a\"}]},\"type\":\"ConnectorPlacement.EquallySpacedConnector\",\"uuid\":\"a2ca7259-7cd6-4f5b-b082-7ba40fce56a8\"}],\"packageUris\":[\"http://schema.mathworks.com/mf0/Connector/R2020b\"],\"version\":\"1.0\"}"
  m_data_tdata : Outport
  m_data_tvalid : Outport  Port=2
  s_data_tready : Outport  Port=3
  wires:
  log2/1(m_data_tvalid) -> Delay2/1
  FIR Compiler 7.2/2 -> exp/1(s_data_tvalid)
  exp/3(s_data_tready) -> FIR Compiler 7.2/3, Delay2/2, CMult1/2, log2/3(m_data_tready)
  s_data_tvalid/1 -> Inverter/1
  FIR_polyphase_decimator_2/2 -> Logical1/2, Delay/1
  FIR_polyphase_decimator_2/3 -> Delay1/1
  homo_m_data_tdata/1 -> m_data_tdata/1
  Inverter/1 -> log2/2(s_data_tvalid)
  log2/3(s_data_tready) -> s_data_tready/1
  exp/2(m_data_tdata) -> FIR_polyphase_decimator_2/2
  s_data_tdata/1 -> log2/1(s_data_tdata)
  log2/2(m_data_tdata) -> CMult1/1
  FIR Compiler 7.2/3 -> exp/2(s_data_tdata)
  CMult1/1 -> FIR Compiler 7.2/2
  Delay2/1 -> FIR Compiler 7.2/1
  Inverter4/1 -> Counter2/1
  Counter2/1 -> Relational8/1
  Constant12/1 -> Relational8/2
  Logical/1 -> Logical8/2, exp/3(m_data_tready), FIR_polyphase_decimator_2/3
  m_data_tready/1 -> Logical1/1, Logical/1, Inverter4/1
  homo_m_data_tvalid/1 -> m_data_tvalid/1
  Logical8/1 -> homo_m_data_tvalid/1, Counter2/2
  exp/1(m_data_tvalid) -> FIR_polyphase_decimator_2/1
  Relational8/1 -> Logical/2
  FIR_polyphase_decimator_2/1 -> Terminator/1
  FIR Compiler 7.2/1 -> Terminator1/1
  Constant/1 -> Relational/2
  Relational/1 -> Register1/2, Register/2, Logical1/3
  Counter/1 -> Relational/1
  Logical1/1 -> Counter/1
  Delay/1 -> Register/1
  Register/1 -> Logical8/1
  Delay1/1 -> Register1/1
  Register1/1 -> homo_m_data_tdata/1
